simulink model "lotker"  (R2024b)
settings: Solver=VariableStepAuto  StartTime=0.0  StopTime=10.0  MaxStep=0.01  RelTol=1e-3
values from neighbouring files (symbols this model uses):
  a = 0.6    [model_lotkera.m]
  b = 0.4    [model_lotkera.m]
  P_0 = P_0_n(j)    [model_lotkera.m]
  r_sp = 1    [model_lotkera.m]
  r_vv = r_vv_n(i)    [model_lotkera.m]
  V_0 = V_0_n(j)    [model_lotkera.m]
settings Model: Creator=userbrigh  LastModifiedBy=userbrigh

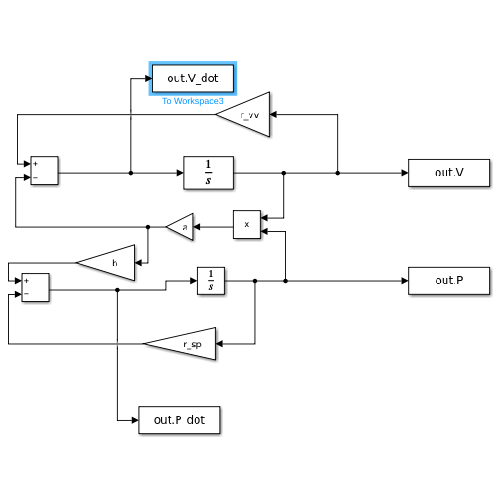
[thumbnail: Simulink's stored preview of the top-level diagram]
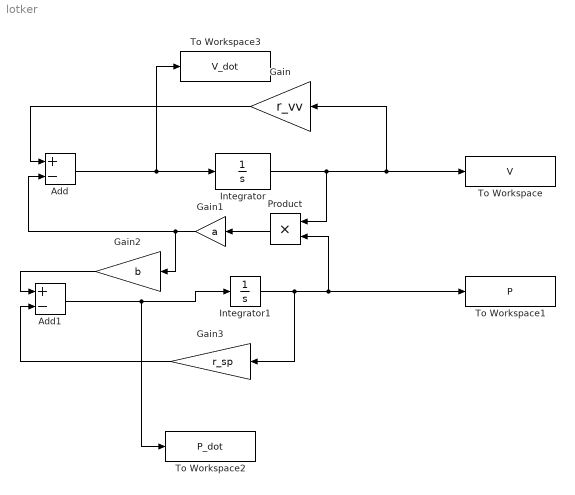
== system lotker ==
  Add : Sum  Inputs=+-
  Add1 : Sum  Inputs=+-
  Gain : Gain  Gain=r_vv
  Gain1 : Gain  Gain=a
  Gain2 : Gain  Gain=b
  Gain3 : Gain  Gain=r_sp
  Integrator : Integrator  InitialCondition=V_0
  Integrator1 : Integrator  InitialCondition=P_0
  Product : Product
  To Workspace : ToWorkspace  VariableName=V  SampleTime=-1
  To Workspace1 : ToWorkspace  VariableName=P  SampleTime=-1
  To Workspace2 : ToWorkspace  VariableName=P_dot  SampleTime=-1
  To Workspace3 : ToWorkspace  VariableName=V_dot  SampleTime=-1
  wires:
  Integrator1/1 -> Gain3/1, Product/2, To Workspace1/1
  Integrator/1 -> Product/1, To Workspace/1, Gain/1
  Gain/1 -> Add/1
  Product/1 -> Gain1/1
  Gain1/1 -> Gain2/1, Add/2
  Add/1 -> To Workspace3/1, Integrator/1
  Gain2/1 -> Add1/1
  Gain3/1 -> Add1/2
  Add1/1 -> Integrator1/1, To Workspace2/1
